simulink model "IEEE_9bus"  (R2023b)
settings: Solver=ode23tb  StartTime=0.0  StopTime=1  FixedStep=Ts  RelTol=1e-3
values from neighbouring files (symbols this model uses):
  N = 1    [IEEE_9bus_calc.m]
  Ts = 50e-6    (= 5e-05)    [IEEE_9bus_calc.m]
  Ws = 2*pi*f    (= 376.991118431)    [IEEE_9bus_calc.m]
undefined symbols (not defined in the file or in its folder): D1, Delta, DiscIntNeverNeededParam, SM, SYS
libraries: spsLoadFlowBusLib x9, spsabctodq0Lib x7, spsThreePhasePISectionLineLib x6, spsExcitationSystemLib x6, spsGenericPowerSystemStabilizerLib x6, spsHydraulicTurbineandGovernorLib x6, spsMultiBandPowerSystemStabilizerLib x6, spsThreePhaseVIMeasurementLib x5, spsThreePhaseSeriesRLCLoadLib x4, DQN_Lib x3, spsGroundLib x3, spsThreePhaseParallelRLCBranchLib x3
(part 2 of 3)

== system IEEE_9bus/ABsel ==
  In1 : Inport
  Demux : Demux  Outputs=3
  Mux : Mux  Inputs=3
  Subtract : Sum  Inputs=--
  Out1 : Outport
  wires:
  In1/1 -> Demux/1
  Demux/1 -> Subtract/1, Mux/1
  Mux/1 -> Out1/1
  Demux/2 -> Subtract/2, Mux/2
  Subtract/1 -> Mux/3

== system IEEE_9bus/ABsel1 ==
  In1 : Inport
  Demux : Demux  Outputs=3
  Mux : Mux  Inputs=3
  Subtract : Sum  Inputs=--
  Out1 : Outport
  wires:
  In1/1 -> Demux/1
  Demux/1 -> Subtract/1, Mux/1
  Mux/1 -> Out1/1
  Demux/2 -> Subtract/2, Mux/2
  Subtract/1 -> Mux/3

== system IEEE_9bus/ABsel2 ==
  In1 : Inport
  Demux : Demux  Outputs=3
  Mux : Mux  Inputs=3
  Subtract : Sum  Inputs=--
  Out1 : Outport
  wires:
  In1/1 -> Demux/1
  Demux/1 -> Subtract/1, Mux/1
  Mux/1 -> Out1/1
  Demux/2 -> Subtract/2, Mux/2
  Subtract/1 -> Mux/3

== system IEEE_9bus/ABsel3 ==
  In1 : Inport
  Demux : Demux  Outputs=3
  Mux : Mux  Inputs=2
  Subtract : Sum  Inputs=+-
  Subtract1 : Sum  Inputs=+-
  Out1 : Outport
  wires:
  In1/1 -> Demux/1
  Mux/1 -> Out1/1
  Demux/1 -> Subtract/1
  Demux/2 -> Subtract1/1, Subtract/2
  Subtract/1 -> Mux/1
  Subtract1/1 -> Mux/2
  Demux/3 -> Subtract1/2

== system IEEE_9bus/ABsel4 ==
  In1 : Inport
  Demux : Demux  Outputs=2
  Mux : Mux  Inputs=3
  Subtract : Sum  Inputs=--
  Out1 : Outport
  wires:
  In1/1 -> Demux/1
  Demux/1 -> Subtract/1, Mux/1
  Mux/1 -> Out1/1
  Demux/2 -> Mux/2, Subtract/2
  Subtract/1 -> Mux/3

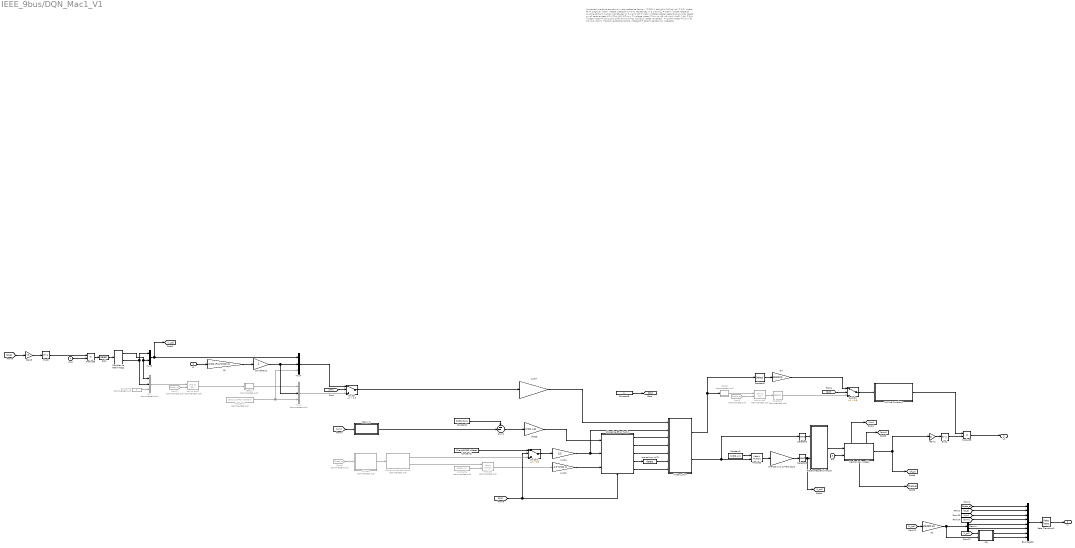
== system IEEE_9bus/DQN_Mac1_V1 ==
  note: Implement  machine equations in rotor reference frame:
      |   v = [R]*i + dphi/dt + [W]*phi
      | phi = [L]*i
      |
      | where:
      | [R] = diagonal matrix (nState,nState)of winding resistances in d q axis
      | [L] = matrix (nSate,nState)of winding self and mutual inductances in d q axis
      | [W] = matrix (nState,nState) depending on rotor speed wr,
      |       all zeros except W(1,2)=wr  W(2,1)=-wr
      |
      |   v = voltage vector      = [vq   vd   vfd   vkd   vkq1   (vkq2)  ]'
      | phi = flux linkage vector = [phiq phid phifd phikd phikq1 (phikq2)]' (state variables)
      |   i = current vector      = [iq   id   ifd   ikd   ikq1   (ikq2)  ]'
      |
      | if RotorType=Salient-Pole, nState=5
      | if RotorType=Round,        nState=6
  Vs_C : Inport
  Vf : Inport  Port=2
  Pm : Inport  Port=3
  1_Vb1 : Gain  Gain=-0.5*SMRD.Ib  SaturateOnIntegerOverflow=on  OutDataTypeStr=Inherit: Same as input  ParamDataTypeStr=Inherit: Same as input
  1_Vb4 : Gain  Gain=1/3  SaturateOnIntegerOverflow=on  OutDataTypeStr=Inherit: Same as input  ParamDataTypeStr=Inherit: Same as input
  1_Vb7 : Gain  Gain=SMRD.web/SMRD.Vb  SaturateOnIntegerOverflow=on  OutDataTypeStr=Inherit: Same as input  ParamDataTypeStr=Inherit: Same as input
  ABsel2 : Subsystem  Commented=on
  ABsel3 : Subsystem  Commented=on
  Bus Creator : BusCreator  Inputs=8
  Complex to Real-Imag1 : ComplexToRealImag
  Constant : Constant  Commented=on  Value=zeros(1,SMRD.nState-3)
  Constant1 : Constant  Value=SMRD.RLinv
  Constant2 : Constant  Value=3*eye(SMRD.nState)
  Constant4 : Constant  Commented=on  Value=SMRD.Linv
  Constant5 : Constant  Commented=on  Value=0
  Constant7 : Constant  Value=SMRD.Linv
  Constant8 : Constant
  Demux : Demux  Outputs=2
  Discretize BE or Tustin : Subsystem
      settings: PortSchema="{\"entries\":[{\"content\":{\"sides\":[{\"content\":{\"connectorIds\":[\"In1\",\"In2\",\"In3\"]},\"type\":\"ConnectorPlacement.EquallySpacedRectSide\",\"uuid\":\"a6b8bc68-dacc-495a-bf9e-1715fd4ce50f\"},{\"content\":{\"connectorIds\":[\"Out1\",\"Out2\",\"Out3\",\"Out4\",\"Out5\"],\"side\":\"RIGHT\"},\"type\":\"ConnectorPlacement.EquallySpacedRectSide\",\"uuid\":\"950ac892-f5e8-4081-8a8f-99bab3dfce2c\"},{\"content\":{\"side\":\"TOP\"},\"type\":\"ConnectorPlacement.EquallySpacedRectSide\",\"uuid\":\"9af2ed0d-ba89-43cd-9977-15872ca13b39\"},{\"content\":{\"connectorIds\":[\"In4\"],\"side\":\"BOTTOM\"},\"type\":\"ConnectorPlacement.EquallySpacedRectSide\",\"uuid\":\"e70e144b-23c4-40ad-9fe1-8550fd976efc\"}]},\"type\":\"ConnectorPlacement.EquallySpacedConnector\",\"uuid\":\"50b9889c-6d2c-45b1-ad8f-98a7760fa0a3\"}],\"packageUris\":[\"http://schema.mathworks.com/mf0/Connector/R2020b\"],\"version\":\"1.0\"}"
  Electromagnetic Torque : Subsystem
  Exp2 : Math
  Exp3 : Math
  From3 : From  Commented=on  GotoTag=theta_e
  From5 : From  Commented=on  GotoTag=theta_e
  From8 : From  Commented=on  GotoTag=theta_e
  Gain2 : Gain  Gain=1i
  Gain3 : Gain  Gain=-1i
  Ihistory_Flux : Subsystem
  MATLAB Function2 : MATLAB Function  TreatAsAtomicUnit=on  mask{N=SMRD.N}
      mask prompts: N "Harmonic order:"
  Matrix W : Subsystem
      settings: LibrarySourceBlock=spsSynchronousMachineModel/Discrete robust/Matrix W
  Mechanical model1 : Subsystem
      settings: LibrarySourceBlock=spsSynchronousMachineModel/Discrete Pm input trapezoidal  PortSchema="{\"entries\":[{\"content\":{\"sides\":[{\"content\":{\"connectorIds\":[\"In1\",\"In2\"]},\"type\":\"ConnectorPlacement.EquallySpacedRectSide\",\"uuid\":\"2381534f-5abc-4a8d-aa04-ab974f15f8a1\"},{\"content\":{\"connectorIds\":[\"Out1\"],\"side\":\"RIGHT\"},\"type\":\"ConnectorPlacement.EquallySpacedRectSide\",\"uuid\":\"4b91f832-d568-486f-91ee-7f5a07d19f05\"},{\"content\":{\"connectorIds\":[\"Out3\",\"Out4\"],\"side\":\"TOP\"},\"type\":\"ConnectorPlacement.EquallySpacedRectSide\",\"uuid\":\"94f23016-8fd9-49f0-81e0-4b44cc2bc22e\"},{\"content\":{\"connectorIds\":[\"Out2\"],\"side\":\"BOTTOM\"},\"type\":\"ConnectorPlacement.EquallySpacedRectSide\",\"uuid\":\"caf2a10e-4688-4978-a259-17b5afc46c0a\"}]},\"type\":\"ConnectorPlacement.EquallySpacedConnector\",\"uuid\":\"5998548e-4f7b-436e-b4ae-37de4e285cc4\"}],\"packageUris\":[\"http://schema.mathworks.com/mf0/Connector/R2020b\"],\"version\":\"1.0\"}"
  Mux : Mux  Commented=on  Inputs=3
  Mux1 : Mux  Commented=on  Inputs=[2 1 SMRD.nState-3]
  Mux3 : Mux  Inputs=2
  Mux4 : Mux  Inputs=[2 1 SMRD.nState-3]
  N1 : Gain  Gain=SMRD.Vfnp*SMRD.Vb  SaturateOnIntegerOverflow=on  OutDataTypeStr=Inherit: Same as input  ParamDataTypeStr=Inherit: Same as input
  N2 : Gain  Gain=1/SMRD.Vb  SaturateOnIntegerOverflow=on  OutDataTypeStr=Inherit: Same as input  ParamDataTypeStr=Inherit: Same as input
  PQ : Subsystem  AncestorBlock=spsSynchronousMachineModel/Discrete robust/Machine Measurements/PQ
  Product2 : Product  Multiplication=Matrix(*)  SaturateOnIntegerOverflow=on  OutDataTypeStr=Inherit: Same as first input
  Product4 : Product  Commented=on  Multiplication=Matrix(*)  SaturateOnIntegerOverflow=on  OutDataTypeStr=Inherit: Same as first input
  Product5 : Product
  Product6 : Product
  Rate Transition2 : RateTransition  Deterministic=off  OutPortSampleTime=Ts
  SM.VfGain1 : Gain
  Sel1 : Selector  NumberOfDimensions=2  InputPortWidth=3  IndexOptions=Index vector (dialog),Index vector (dialog)  Indices=1,2  OutputSizes=1
  Selector1 : Selector  Commented=on  InputPortWidth=3  IndexOptions=Index vector (dialog)  Indices=[1 2]  OutputSizes=1
  Selector2 : Selector  InputPortWidth=SMRD.nState  IndexOptions=Index vector (dialog)  Indices=[1 2]  OutputSizes=1
  Selector3 : Selector  InputPortWidth=SMRD.nState  IndexOptions=Index vector (dialog)  Indices=[1 2]  OutputSizes=1
  Selector5 : Selector  InputPortWidth=2  IndexOptions=Index vector (dialog)  Indices=[2 1]  OutputSizes=1
  Sum1 : Sum  Inputs=--|  SaturateOnIntegerOverflow=on
  Switch : Switch  Criteria=u2 > Threshold  Threshold=0.5  SaturateOnIntegerOverflow=off  InputSameDT=off
  Switch1 : Switch  Criteria=u2 > Threshold  Threshold=0.5  SaturateOnIntegerOverflow=off  InputSameDT=off
  Switch3 : Switch  Criteria=u2 > Threshold  Threshold=0.5  SaturateOnIntegerOverflow=off  InputSameDT=off
  abc to dq transformation : Subsystem  Commented=on
      settings: LibrarySourceBlock=|
      | spsSynchronousMachineModel/Discrete robust/abc to dq
      | transformation
  abc to dq0 : spsabctodq0Lib/abc to dq0  Commented=on  Alignment=90 degrees behind phase A axis
  change Iq Id current signs : Gain  Gain=SMRD.IqdSign
  dq0 to abc1 : spsdq0toabcLib/dq0 to abc  Commented=on  Alignment=90 degrees behind phase A axis
  ib4 : Gain  Gain=SMRD.Ib  SaturateOnIntegerOverflow=on  OutDataTypeStr=Inherit: Same as input  ParamDataTypeStr=Inherit: Same as input
  last column of D : Selector  NumberOfDimensions=2  InputPortWidth=3  IndexOptions=Index vector (dialog),Index vector (dialog)  Indices=[1:SMRD.nState],3  OutputSizes=1,1
  sin,cos : Subsystem  Commented=on
      settings: LibrarySourceBlock=spsSynchronousMachineModel/Discrete robust/sin,cos
  wbase : Gain  Gain=SMRD.web
  I_C : Outport  VectorParamsAs1DForOutWhenUnconnected=off
  m : Outport  Port=2  VectorParamsAs1DForOutWhenUnconnected=off
  wires:
  Vs_C/1 -> Product6/2  "vd,vq"
  sin,cos/1(sin,cos) -> abc to dq transformation/1(sin,cos)
  1_Vb1/1 -> Discretize BE or Tustin/3(C)
  last column of D/1 -> Ihistory_Flux/6(D(:,3))
  Discretize BE or Tustin/1(Ad) -> Ihistory_Flux/3(Ad)
  Discretize BE or Tustin/4(Dd) -> last column of D/1
  Electromagnetic Torque/1(Te) -> Mechanical model1/1(Te)
  Product2/1 -> change Iq Id current signs/1
  wbase/1 -> Discretize BE or Tustin/1(A)
  Discretize BE or Tustin/5(inv(I_Ts/2*A)) -> Ihistory_Flux/7(inv())
  Discretize BE or Tustin/2(Bd) -> Ihistory_Flux/4(Bd)
  Constant4/1 -> Product4/2  "Linv"
  Matrix W/1("[W]") -> Sum1/2
  Sum1/1 -> wbase/1  "A"
  Product4/1 -> 1_Vb1/1
  Ihistory_Flux/2(phi) -> Product2/2, Selector2/1
  Mechanical model1/2(theta_e) -> [theta_e]
  Mechanical model1/3(we) -> [wm]
  Pm/1 -> Mechanical model1/2(input)
  Constant7/1 -> Product2/1  "Linv"
  Constant2/1 -> Switch1/1
  ABsel3/1(Out1) -> Mux1/1
  Mux1/1 -> Switch/3  "u"
  Constant1/1 -> Sum1/1
  Vf/1 -> N1/1  "Vfd"
  Constant/1 -> Mux1/3, Mux4/3
  SM.VfGain1/1 -> Mux4/2, Mux1/2
  Mux4/1 -> Switch/1  "u"
  N1/1 -> SM.VfGain1/1  "Vfd"
  dq0 to abc1/1 -> ABsel3/1(v)
  abc to dq transformation/2(Ti (2x2)) -> Product4/1
  Switch1/1 -> 1_Vb4/1  "u"
  Ihistory_Flux/1(Ihyst) -> Selector5/1, ABsel2/1(v)  "I(k) = Linv*phi"
  MATLAB Function2/1(Vs_c) -> Product5/1
  Exp2/1 -> Product5/2
  Gain2/1 -> Exp2/1
  Switch/1 -> 1_Vb7/1
  Gain3/1 -> Exp3/1
  [dt_e] -> Gain3/1
  Product6/1 -> Sel1/1
  Exp3/1 -> Product6/1
  Sel1/1 -> Complex to Real-Imag1/1
  Mechanical model1/1(dtheta_e) -> [dt_e], Gain2/1
  Complex to Real-Imag1/2 -> Mux3/1, Mux/2
  Complex to Real-Imag1/1 -> Mux/1, Mux3/2
  Mux3/1 -> [v_qd], Mux4/1
  Switch3/1 -> MATLAB Function2/1(Vdq_vec)
  Mux/1 -> dq0 to abc1/1
  From3/1 -> dq0 to abc1/2
  Constant5/1 -> Mux/3
  1_Vb7/1 -> Ihistory_Flux/1(u)  "u"
  [SW] -> Switch/2
  Constant8/1 -> [SW]
  [SW] -> Switch1/2, Discretize BE or Tustin/4(SW)
  abc to dq transformation/1(Tv (nx3)) -> Switch1/3
  Selector1/1 -> Switch3/3  "Linv"
  [SW] -> Switch3/2
  Selector5/1 -> ib4/1
  abc to dq0/1 -> Selector1/1
  ABsel2/1(I) -> abc to dq0/1
  ib4/1 -> Switch3/1
  From5/1 -> abc to dq0/2
  Product5/1 -> I_C/1
  1_Vb4/1 -> Ihistory_Flux/2(B), Discretize BE or Tustin/2(B)
  [wm] -> Matrix W/1(wr)
  From8/1 -> sin,cos/1(theta)
  Discretize BE or Tustin/3(Cd) -> Ihistory_Flux/5(Cd)
  Bus Creator/1 -> Rate Transition2/1
  [theta_e] -> Bus Creator/1  "Rotor electrical angle  theta (rad)"
  [dt_e] -> Bus Creator/2  "Rotor angle deviation  d_theta (rad)"
  [wm] -> Bus Creator/3  "Rotor speed  wm  (pu)"
  Rate Transition2/1 -> m/1
  [v_qd] -> N2/1
  [i_qd] -> PQ/1(Iqd)
  PQ/1(Peo) -> Bus Creator/7  "Output active power   Peo (pu)"
  PQ/2(Qeo) -> Bus Creator/8  "Output reactive power  Qeo (pu)"
  Mechanical model1/4(dwe) -> [dwm]
  [dwm] -> Bus Creator/4  "Rotor speed deviation  dw (pu)"
  change Iq Id current signs/1 -> Selector3/1
  Selector3/1 -> [i_qd], Electromagnetic Torque/2(iqd)
  Selector2/1 -> Electromagnetic Torque/1(phiqd)
  N2/1 -> PQ/2(Vqd), Demux/1  "Vfd"
  Demux/1 -> Bus Creator/5  "Stator voltage  vq (pu)"
  Demux/2 -> Bus Creator/6  "Stator voltage  vd (pu)"

== system IEEE_9bus/Demux_DQNc_Mat ==
  In1 : Inport
  Sel1 : Selector  NumberOfDimensions=2  InputPortWidth=3  IndexOptions=Index vector (dialog),Select all  Indices=1:3, 1  OutputSizes=1
  Sel2 : Selector  NumberOfDimensions=2  InputPortWidth=3  IndexOptions=Index vector (dialog),Select all  Indices=4:6, 1  OutputSizes=1
  Sel3 : Selector  NumberOfDimensions=2  InputPortWidth=3  IndexOptions=Index vector (dialog),Select all  Indices=7:9, 1  OutputSizes=1
  Out1 : Outport
  Out2 : Outport  Port=2
  Out3 : Outport  Port=3
  wires:
  In1/1 -> Sel1/1, Sel2/1, Sel3/1
  Sel1/1 -> Out1/1
  Sel2/1 -> Out2/1
  Sel3/1 -> Out3/1

== system IEEE_9bus/Demux_DQNc_Mat2 ==
  In1 : Inport
  Sel1 : Selector  NumberOfDimensions=2  InputPortWidth=3  IndexOptions=Index vector (dialog),Select all  Indices=1:3, 1  OutputSizes=1
  Sel2 : Selector  NumberOfDimensions=2  InputPortWidth=3  IndexOptions=Index vector (dialog),Select all  Indices=4:6, 1  OutputSizes=1
  Sel3 : Selector  NumberOfDimensions=2  InputPortWidth=3  IndexOptions=Index vector (dialog),Select all  Indices=7:9, 1  OutputSizes=1
  Out1 : Outport
  Out2 : Outport  Port=2
  Out3 : Outport  Port=3
  wires:
  In1/1 -> Sel1/1, Sel2/1, Sel3/1
  Sel1/1 -> Out1/1
  Sel2/1 -> Out2/1
  Sel3/1 -> Out3/1

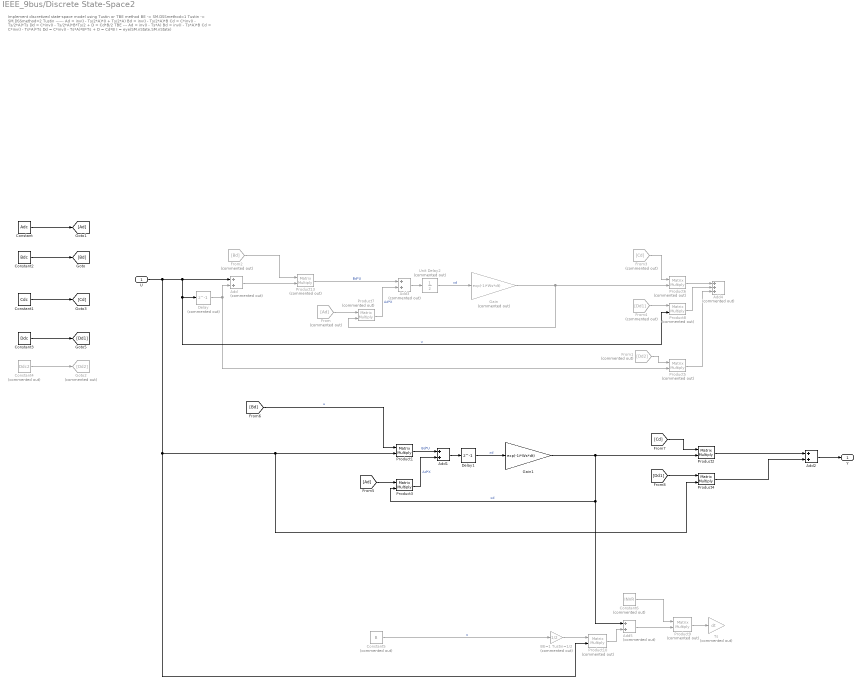
== system IEEE_9bus/Discrete State-Space2 ==
  note: Implement discretized state-space model using Tustin or TBE method
      |
      | BE      -> SM.DSSmethod=1
      | Tustin  -> SM.DSSmethod=2
      |
      |
      | Tustin
      | ------
      | Ad = inv(I - Ts/2*A)*(I + Ts/2*A)
      | Bd = inv(I - Ts/2*A)*B
      | Cd = C*inv(I - Ts/2*A)*Ts
      | Dd = C*inv(I - Ts/2*A)*B*Ts/2  + D  =  Cd*B/2
      |
      | TBE
      | ---
      | Ad = inv(I - Ts*A)
      | Bd = inv(I - Ts*A)*B
      | Cd = C*inv(I - Ts*A)*Ts
      | Dd = C*inv(I - Ts*A)*B*Ts  + D  =  Cd*B
      |
      | I = eye(SM.nState,SM.nState)
  U : Inport
  Add : Sum  Commented=on
  Add1 : Sum
  Add2 : Sum
  Add3 : Sum  Commented=on
  Add4 : Sum  Commented=on  Inputs=+++
  Add5 : Sum  Commented=on
  BE=1 Tustin=1/2 : Gain  Commented=on  Gain=1/2
  Constant : Constant  Value=Adc
  Constant1 : Constant  Value=Cdc
  Constant2 : Constant  Value=Bdc
  Constant3 : Constant  Value=Ddc
  Constant4 : Constant  Commented=on  Value=Ddc2
  Constant5 : Constant  Commented=on  Value=B
  Constant6 : Constant  Commented=on  Value=INVR
  Delay : Delay  Commented=on  DelayLength=1  SampleTime=dt
  Delay1 : Delay  DelayLength=1  InitialCondition=InitVec_c  SampleTime=dt
  From : From  Commented=on  GotoTag=Ad
  From1 : From  Commented=on  GotoTag=Dd2
  From2 : From  Commented=on  GotoTag=Bd
  From3 : From  Commented=on  GotoTag=Cd
  From4 : From  Commented=on  GotoTag=Dd1
  Gain : Gain  Commented=on  Gain=exp(-1i*Ws*dt)
  Gain1 : Gain  Gain=exp(-1i*Ws*dt)
  Goto2 : Goto  Commented=on  GotoTag=Dd2
  Product{1..4} (4 alike) : Product  Multiplication=Matrix(*)  SaturateOnIntegerOverflow=on  OutDataTypeStr=Inherit: Same as first input
  Product{5..10,13} (7 alike) : Product  Commented=on  Multiplication=Matrix(*)  SaturateOnIntegerOverflow=on  OutDataTypeStr=Inherit: Same as first input
  Ts : Gain  Commented=on  Gain=dt  SaturateOnIntegerOverflow=on  OutDataTypeStr=Inherit: Same as input  ParamDataTypeStr=Inherit: Same as input
  Unit Delay2 : UnitDelay  Commented=on  InitialCondition=(Cdc\InitVec_c)  SampleTime=dt  HasFrameUpgradeWarning=on
  Y : Outport
  wires:
  Constant4/1 -> Goto2/1
  Constant3/1 -> [Dd1]
  Constant1/1 -> [Cd]
  Constant2/1 -> [Bd]
  Constant/1 -> [Ad]
  From1/1 -> Product5/1
  Product5/1 -> Add4/3
  Product8/1 -> Add4/2
  From/1 -> Product7/1
  From4/1 -> Product8/1
  From2/1 -> Product13/1
  Product13/1 -> Add3/1  "Bd*U"
  Product7/1 -> Add3/2  "Ad*X"
  Add/1 -> Product13/2
  Product6/1 -> Add4/1
  Unit Delay2/1 -> Gain/1  "xd"
  From3/1 -> Product6/1
  Delay/1 -> Product5/2, Add/2
  Add3/1 -> Unit Delay2/1
  Gain/1 -> Product7/2, Product6/2
  Product1/1 -> Add1/1  "Bd*U"
  Product2/1 -> Add2/1
  [Dd1] -> Product4/1
  Product4/1 -> Add2/2
  [Bd] -> Product1/1  "u"
  Product3/1 -> Add1/2  "Ad*X"
  [Cd] -> Product2/1
  Delay1/1 -> Gain1/1  "xd"
  Add1/1 -> Delay1/1
  [Ad] -> Product3/1
  Constant5/1 -> BE=1 Tustin=1/2/1  "u"
  Product9/1 -> Ts/1
  Constant6/1 -> Product9/1
  Add5/1 -> Product9/2
  U/1 -> Product10/2, Product4/2, Product1/2, Add/1, Product8/2, Delay/1  "u"
  BE=1 Tustin=1/2/1 -> Product10/1
  Product10/1 -> Add5/2
  Gain1/1 -> Product3/2, Add5/1, Product2/2  "xd"
  Add2/1 -> Y/1

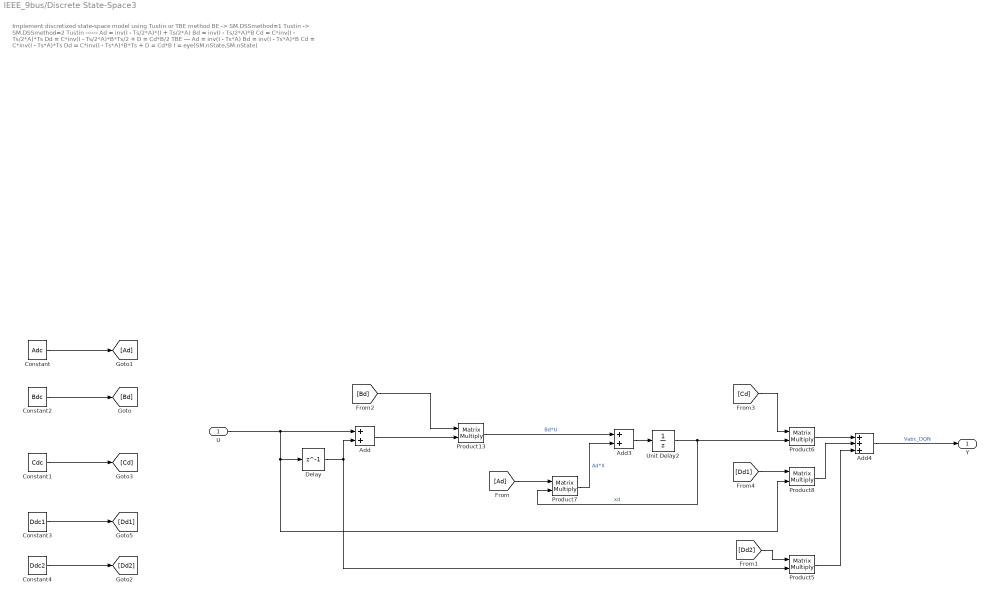
== system IEEE_9bus/Discrete State-Space3 ==
  note: Implement discretized state-space model using Tustin or TBE method
      |
      | BE      -> SM.DSSmethod=1
      | Tustin  -> SM.DSSmethod=2
      |
      |
      | Tustin
      | ------
      | Ad = inv(I - Ts/2*A)*(I + Ts/2*A)
      | Bd = inv(I - Ts/2*A)*B
      | Cd = C*inv(I - Ts/2*A)*Ts
      | Dd = C*inv(I - Ts/2*A)*B*Ts/2  + D  =  Cd*B/2
      |
      | TBE
      | ---
      | Ad = inv(I - Ts*A)
      | Bd = inv(I - Ts*A)*B
      | Cd = C*inv(I - Ts*A)*Ts
      | Dd = C*inv(I - Ts*A)*B*Ts  + D  =  Cd*B
      |
      | I = eye(SM.nState,SM.nState)
  U : Inport
  Add : Sum
  Add3 : Sum
  Add4 : Sum  Inputs=+++
  Constant : Constant  Value=Adc
  Constant1 : Constant  Value=Cdc
  Constant2 : Constant  Value=Bdc
  Constant3 : Constant  Value=Ddc1
  Constant4 : Constant  Value=Ddc2
  Delay : Delay  DelayLength=1  SampleTime=Ts
  Product{5..8,13} (5 alike) : Product  Multiplication=Matrix(*)  SaturateOnIntegerOverflow=on  OutDataTypeStr=Inherit: Same as first input
  Unit Delay2 : UnitDelay  InitialCondition=InitVec_c  SampleTime=dt  HasFrameUpgradeWarning=on
  Y : Outport
  wires:
  Constant4/1 -> [Dd2]
  Constant3/1 -> [Dd1]
  Constant1/1 -> [Cd]
  Constant2/1 -> [Bd]
  Constant/1 -> [Ad]
  Add4/1 -> Y/1  "Vabc_DQN"
  [Dd2] -> Product5/1
  Product5/1 -> Add4/3
  Product8/1 -> Add4/2
  [Ad] -> Product7/1
  [Dd1] -> Product8/1
  U/1 -> Add/1, Product8/2, Delay/1
  [Bd] -> Product13/1
  Product13/1 -> Add3/1  "Bd*U"
  Product7/1 -> Add3/2  "Ad*X"
  Add/1 -> Product13/2
  Product6/1 -> Add4/1
  Unit Delay2/1 -> Product7/2, Product6/2  "xd"
  [Cd] -> Product6/1
  Delay/1 -> Product5/2, Add/2
  Add3/1 -> Unit Delay2/1

== system IEEE_9bus/MatMux1 ==
  In1 : Inport
  In2 : Inport  Port=2
  In3 : Inport  Port=3
  Mux : Concatenate  NumInputs=3  Mode=Multidimensional array
  Out1 : Outport
  wires:
  In1/1 -> Mux/1
  In2/1 -> Mux/2
  In3/1 -> Mux/3
  Mux/1 -> Out1/1

== system IEEE_9bus/MatMux2 ==
  In1 : Inport
  In2 : Inport  Port=2
  In3 : Inport  Port=3
  Mux : Concatenate  NumInputs=3  Mode=Multidimensional array
  Out1 : Outport
  wires:
  In1/1 -> Mux/1
  In2/1 -> Mux/2
  In3/1 -> Mux/3
  Mux/1 -> Out1/1

== system IEEE_9bus/MatMux3 ==
  In1 : Inport
  In2 : Inport  Port=2
  In3 : Inport  Port=3
  Mux : Concatenate  NumInputs=3  Mode=Multidimensional array
  Out1 : Outport
  wires:
  In1/1 -> Mux/1
  In2/1 -> Mux/2
  In3/1 -> Mux/3
  Mux/1 -> Out1/1

== system IEEE_9bus/SS_DelayPrediction ==
  in : Inport
  F2 : Gain  Gain=2  SaturateOnIntegerOverflow=on  OutDataTypeStr=Inherit: Same as input  ParamDataTypeStr=Inherit: Same as input
  Sum1 : Sum  Inputs=+-  InputSameDT=on  SaturateOnIntegerOverflow=on  OutDataTypeStr=Inherit: Same as first input
  dw_delay : UnitDelay  InitialCondition=Zpnz_old  SampleTime=Ts  HasFrameUpgradeWarning=on
  dw_predict : UnitDelay  InitialCondition=Zpnz_old  SampleTime=Ts  HasFrameUpgradeWarning=on
  dw : Outport  VectorParamsAs1DForOutWhenUnconnected=off
  wires:
  Sum1/1 -> dw/1
  F2/1 -> Sum1/1
  dw_predict/1 -> Sum1/2
  in/1 -> dw_delay/1
  dw_delay/1 -> F2/1, dw_predict/1

== system IEEE_9bus/Subsystem ==
  cte1 : Constant
  cte2 : Constant  Value=2
  cte3 : Constant  Value=0
  Generic : Outport  VectorParamsAs1DForOutWhenUnconnected=off
  Multiband : Outport  Port=2  VectorParamsAs1DForOutWhenUnconnected=off
  No PSS : Outport  Port=3  VectorParamsAs1DForOutWhenUnconnected=off
  wires:
  cte1/1 -> Generic/1
  cte2/1 -> Multiband/1
  cte3/1 -> No PSS/1

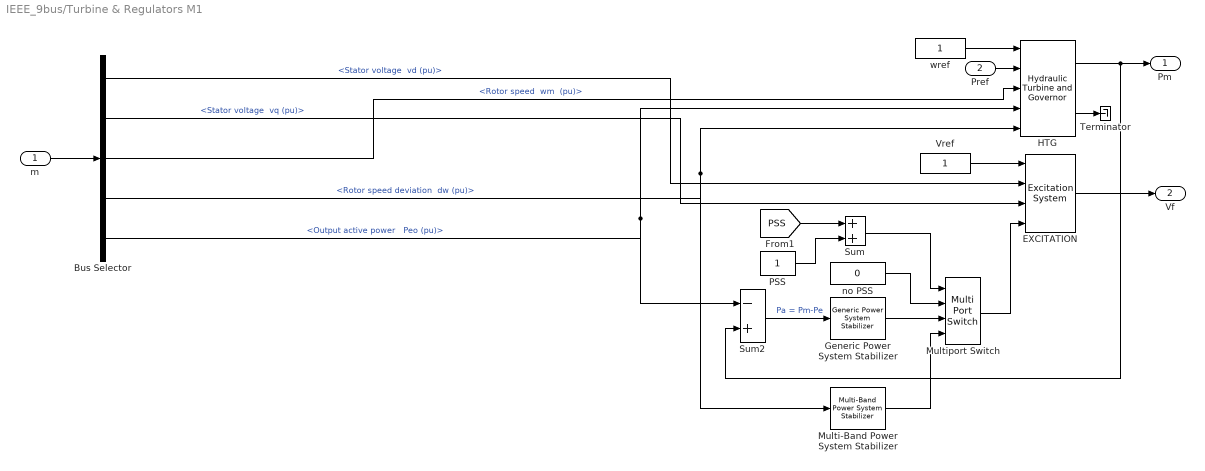
== system IEEE_9bus/Turbine & Regulators M1 ==
  m : Inport
  Pref : Inport  Port=2
  Bus Selector : BusSelector  OutputSignals="dq0 components.Stator voltage  vd (pu),dq0 components.Stator voltage  vq (pu),Mechanical.Rotor speed  wm  (pu),Mechanical.Rotor speed deviation  dw (pu),Output active power   Peo (pu)"
  EXCITATION : spsExcitationSystemLib/Excitation System  tr=20e-3  reg=[ 200, 0.001 ]  exc=[ 1, 0 ]  tgr=[ 0, 0 ]  damp=[ 0.001, 0.1 ]  sat=[ 0, 0 ]  lim="[ 0,  7, 0 ]"  v0=[1 1.5789]
      settings: LibrarySourceBlock=sps_lib/Electrical Machines/Synchronous Machine Control/Excitation System
  Generic Power System Stabilizer : spsGenericPowerSystemStabilizerLib/Generic Power System Stabilizer  Tsensor=15e-3  K=2  Twashout=0.7  Tleadlag1="[60e-3  0.5]"  Tleadlag2=[0 0]  VSlimits=[-0.15 0.15]  Vinit=0  Plot_On=off  MagdB_On=on  FreqRange=logspace(-2,2,500)
      settings: LibrarySourceBlock=|
      | sps_lib/Electrical Machines/Synchronous Machine Control/Generic
      | Power System Stabilizer
  HTG : spsHydraulicTurbineandGovernorLib/Hydraulic Turbine and Governor  sm="[ 10/3  0.07 ]"  gate="[  0.01  0.97518  -0.1  0.1 ]"  reg="[  0.05  1.163  0.105  0  0.01  ]"  hyd="[  0  2.67  ]"  dref=0  po=0.65844
      settings: LibrarySourceBlock=|
      | sps_lib/Electrical Machines/Synchronous Machine Control/Hydraulic Turbine
      | and Governor
  Multi-Band Power System Stabilizer : spsMultiBandPowerSystemStabilizerLib/Multi-Band Power System Stabilizer  OperationMode=Simplified settings  Kg=1.0  GL=[0.025 5]  GI=[0.8 25]  GH=[12.0 145]  GLd=[66 66 9.4]  TcLF=[1.667 2 0 0 0 0 2 2.4 0 0 0 0 1 1]  GId=[66 66 47.6]  TcIF=[1 1 0.25 0.3 0 0 1 1 0.3 0.36 0 0 0 0]  GHd=[66 66 233]  TcHF="[0.01 0.012 0 0 0 0  0.012 0.0144 0 0 0 0 1 1]"  LIM=[.075 .15 .15 .15]  Plot_On=off  MagdB_On=off  FreqRange=logspace(-2,2,500)
      settings: LibrarySourceBlock=|
      | sps_lib/Electrical Machines/Synchronous Machine Control/Multi-Band
      | Power System Stabilizer
  Multiport Switch : MultiPortSwitch  InputSameDT=off
  PSS : Constant
  Sum : Sum  SaturateOnIntegerOverflow=on
  Sum2 : Sum  Inputs=-+  InputSameDT=on  SaturateOnIntegerOverflow=on  OutDataTypeStr=Inherit: Same as first input
  Terminator : Terminator
  Vref : Constant
  no PSS : Constant  Value=0
  wref : Constant
  Pm : Outport  InitialOutput=0  VectorParamsAs1DForOutWhenUnconnected=off
  Vf : Outport  Port=2  InitialOutput=0  VectorParamsAs1DForOutWhenUnconnected=off
  wires:
  PSS/1 -> Sum/2
  [PSS] -> Sum/1
  HTG/2 -> Terminator/1
  Vref/1 -> EXCITATION/1
  m/1 -> Bus Selector/1
  Bus Selector/4 -> Multi-Band Power System Stabilizer/1, HTG/5  "<Rotor speed deviation  dw (pu)>"
  Bus Selector/5 -> Sum2/1, HTG/4  "<Output active power   Peo (pu)>"
  Bus Selector/3 -> HTG/3  "<Rotor speed  wm  (pu)>"
  Pref/1 -> HTG/2
  wref/1 -> HTG/1
  HTG/1 -> Pm/1, Sum2/2
  Bus Selector/2 -> EXCITATION/3  "<Stator voltage  vq (pu)>"
  EXCITATION/1 -> Vf/1
  Bus Selector/1 -> EXCITATION/2  "<Stator voltage  vd (pu)>"
  Sum2/1 -> Generic Power System Stabilizer/1  "Pa = Pm-Pe"
  Generic Power System Stabilizer/1 -> Multiport Switch/3
  Multi-Band Power System Stabilizer/1 -> Multiport Switch/4
  no PSS/1 -> Multiport Switch/2
  Sum/1 -> Multiport Switch/1
  Multiport Switch/1 -> EXCITATION/4

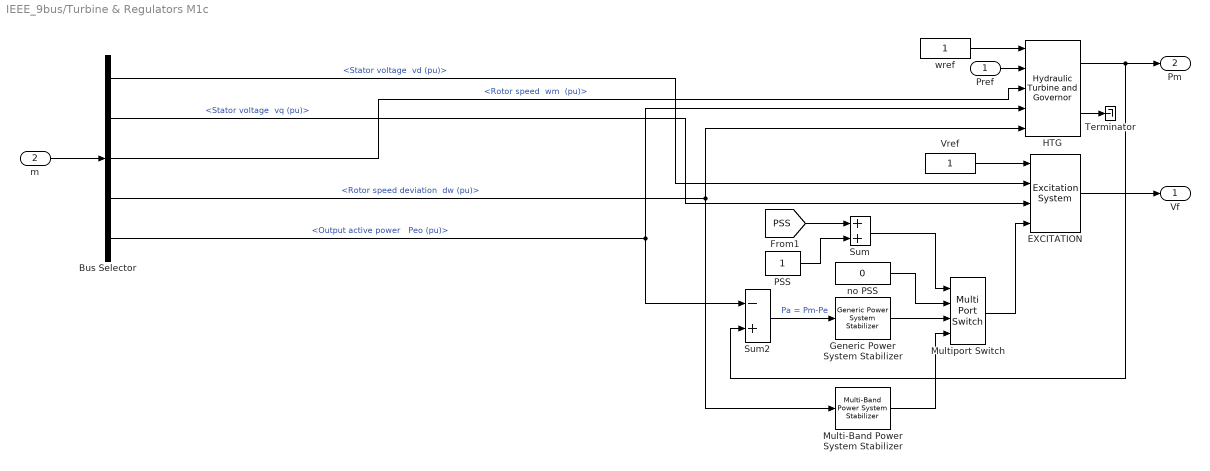
== system IEEE_9bus/Turbine & Regulators M1c ==
  Pref : Inport
  m : Inport  Port=2
  Bus Selector : BusSelector  OutputSignals="Stator voltage  vd (pu),Stator voltage  vq (pu),Rotor speed  wm  (pu),Rotor speed deviation  dw (pu),Output active power   Peo (pu)"
  EXCITATION : spsExcitationSystemLib/Excitation System  tr=20e-3  reg=[ 200, 0.001 ]  exc=[ 1, 0 ]  tgr=[ 0, 0 ]  damp=[ 0.001, 0.1 ]  sat=[ 0, 0 ]  lim="[ 0,  7, 0 ]"  v0=[1 1.5789]
      settings: LibrarySourceBlock=sps_lib/Electrical Machines/Synchronous Machine Control/Excitation System
  Generic Power System Stabilizer : spsGenericPowerSystemStabilizerLib/Generic Power System Stabilizer  Tsensor=15e-3  K=2  Twashout=0.7  Tleadlag1="[60e-3  0.5]"  Tleadlag2=[0 0]  VSlimits=[-0.15 0.15]  Vinit=0  Plot_On=off  MagdB_On=on  FreqRange=logspace(-2,2,500)
      settings: LibrarySourceBlock=|
      | sps_lib/Electrical Machines/Synchronous Machine Control/Generic
      | Power System Stabilizer
  HTG : spsHydraulicTurbineandGovernorLib/Hydraulic Turbine and Governor  sm="[ 10/3  0.07 ]"  gate="[  0.01  0.97518  -0.1  0.1 ]"  reg="[  0.05  1.163  0.105  0  0.01  ]"  hyd="[  0  2.67  ]"  dref=0  po=0.65844
      settings: LibrarySourceBlock=|
      | sps_lib/Electrical Machines/Synchronous Machine Control/Hydraulic Turbine
      | and Governor
  Multi-Band Power System Stabilizer : spsMultiBandPowerSystemStabilizerLib/Multi-Band Power System Stabilizer  OperationMode=Simplified settings  Kg=1.0  GL=[0.025 5]  GI=[0.8 25]  GH=[12.0 145]  GLd=[66 66 9.4]  TcLF=[1.667 2 0 0 0 0 2 2.4 0 0 0 0 1 1]  GId=[66 66 47.6]  TcIF=[1 1 0.25 0.3 0 0 1 1 0.3 0.36 0 0 0 0]  GHd=[66 66 233]  TcHF="[0.01 0.012 0 0 0 0  0.012 0.0144 0 0 0 0 1 1]"  LIM=[.075 .15 .15 .15]  Plot_On=off  MagdB_On=off  FreqRange=logspace(-2,2,500)
      settings: LibrarySourceBlock=|
      | sps_lib/Electrical Machines/Synchronous Machine Control/Multi-Band
      | Power System Stabilizer
  Multiport Switch : MultiPortSwitch  InputSameDT=off
  PSS : Constant
  Sum : Sum  SaturateOnIntegerOverflow=on
  Sum2 : Sum  Inputs=-+  InputSameDT=on  SaturateOnIntegerOverflow=on  OutDataTypeStr=Inherit: Same as first input
  Terminator : Terminator
  Vref : Constant
  no PSS : Constant  Value=0
  wref : Constant
  Vf : Outport  InitialOutput=0  VectorParamsAs1DForOutWhenUnconnected=off
  Pm : Outport  Port=2  InitialOutput=0  VectorParamsAs1DForOutWhenUnconnected=off
  wires:
  PSS/1 -> Sum/2
  [PSS] -> Sum/1
  HTG/2 -> Terminator/1
  Vref/1 -> EXCITATION/1
  m/1 -> Bus Selector/1
  Bus Selector/4 -> HTG/5, Multi-Band Power System Stabilizer/1  "<Rotor speed deviation  dw (pu)>"
  Bus Selector/5 -> HTG/4, Sum2/1  "<Output active power   Peo (pu)>"
  Bus Selector/3 -> HTG/3  "<Rotor speed  wm  (pu)>"
  Pref/1 -> HTG/2
  wref/1 -> HTG/1
  HTG/1 -> Pm/1, Sum2/2
  Bus Selector/2 -> EXCITATION/3  "<Stator voltage  vq (pu)>"
  EXCITATION/1 -> Vf/1
  Bus Selector/1 -> EXCITATION/2  "<Stator voltage  vd (pu)>"
  Sum2/1 -> Generic Power System Stabilizer/1  "Pa = Pm-Pe"
  Generic Power System Stabilizer/1 -> Multiport Switch/3
  Multi-Band Power System Stabilizer/1 -> Multiport Switch/4
  no PSS/1 -> Multiport Switch/2
  Sum/1 -> Multiport Switch/1
  Multiport Switch/1 -> EXCITATION/4

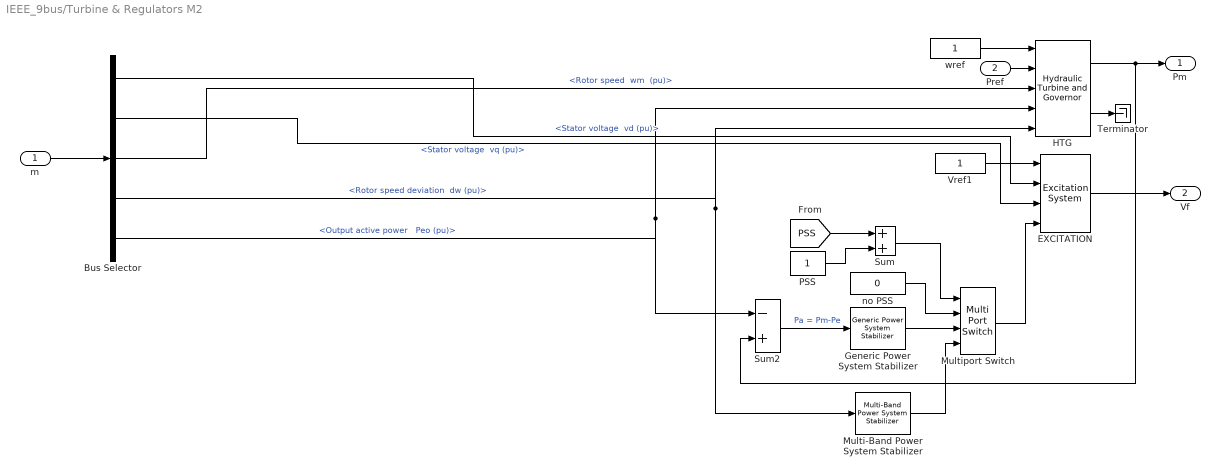
== system IEEE_9bus/Turbine & Regulators M2 ==
  m : Inport
  Pref : Inport  Port=2
  Bus Selector : BusSelector  OutputSignals="dq0 components.Stator voltage  vd (pu),dq0 components.Stator voltage  vq (pu),Mechanical.Rotor speed  wm  (pu),Mechanical.Rotor speed deviation  dw (pu),Output active power   Peo (pu)"
  EXCITATION : spsExcitationSystemLib/Excitation System  tr=20e-3  reg=[ 200, 0.001 ]  exc=[ 1, 0 ]  tgr=[ 0, 0 ]  damp=[ 0.001, 0.1 ]  sat=[ 0, 0 ]  lim="[ 0,  7, 0 ]"  v0=[1 1.5762]
      settings: LibrarySourceBlock=sps_lib/Electrical Machines/Synchronous Machine Control/Excitation System
  Generic Power System Stabilizer : spsGenericPowerSystemStabilizerLib/Generic Power System Stabilizer  Tsensor=15e-3  K=2  Twashout=0.7  Tleadlag1="[60e-3  0.5]"  Tleadlag2=[0 0]  VSlimits=[-0.15 0.15]  Vinit=0  Plot_On=off  MagdB_On=on  FreqRange=logspace(-2,2,500)
      settings: LibrarySourceBlock=|
      | sps_lib/Electrical Machines/Synchronous Machine Control/Generic
      | Power System Stabilizer
  HTG : spsHydraulicTurbineandGovernorLib/Hydraulic Turbine and Governor  sm="[ 10/3  0.07 ]"  gate="[  0.01  0.97518  -0.1  0.1 ]"  reg="[  0.05  1.163  0.105  0  0.01  ]"  hyd="[  0  2.67  ]"  dref=0  po=0.82708
      settings: LibrarySourceBlock=|
      | sps_lib/Electrical Machines/Synchronous Machine Control/Hydraulic Turbine
      | and Governor
  Multi-Band Power System Stabilizer : spsMultiBandPowerSystemStabilizerLib/Multi-Band Power System Stabilizer  OperationMode=Simplified settings  Kg=1.0  GL=[0.025 5]  GI=[0.8 25]  GH=[12.0 145]  GLd=[66 66 9.4]  TcLF=[1.667 2 0 0 0 0 2 2.4 0 0 0 0 1 1]  GId=[66 66 47.6]  TcIF=[1 1 0.25 0.3 0 0 1 1 0.3 0.36 0 0 0 0]  GHd=[66 66 233]  TcHF="[0.01 0.012 0 0 0 0  0.012 0.0144 0 0 0 0 1 1]"  LIM=[.075 .15 .15 .15]  Plot_On=off  MagdB_On=off  FreqRange=logspace(-2,2,500)
      settings: LibrarySourceBlock=|
      | sps_lib/Electrical Machines/Synchronous Machine Control/Multi-Band
      | Power System Stabilizer
  Multiport Switch : MultiPortSwitch  InputSameDT=off
  PSS : Constant
  Sum : Sum  SaturateOnIntegerOverflow=on
  Sum2 : Sum  Inputs=-+  InputSameDT=on  SaturateOnIntegerOverflow=on  OutDataTypeStr=Inherit: Same as first input
  Terminator : Terminator
  Vref1 : Constant
  no PSS : Constant  Value=0
  wref : Constant
  Pm : Outport  InitialOutput=0  VectorParamsAs1DForOutWhenUnconnected=off
  Vf : Outport  Port=2  InitialOutput=0  VectorParamsAs1DForOutWhenUnconnected=off
  wires:
  HTG/2 -> Terminator/1
  Vref1/1 -> EXCITATION/1
  m/1 -> Bus Selector/1
  Bus Selector/4 -> HTG/5, Multi-Band Power System Stabilizer/1  "<Rotor speed deviation  dw (pu)>"
  Bus Selector/3 -> HTG/3  "<Rotor speed  wm  (pu)>"
  Pref/1 -> HTG/2
  wref/1 -> HTG/1
  HTG/1 -> Pm/1, Sum2/2
  Bus Selector/2 -> EXCITATION/3  "<Stator voltage  vq (pu)>"
  EXCITATION/1 -> Vf/1
  Bus Selector/1 -> EXCITATION/2  "<Stator voltage  vd (pu)>"
  Sum2/1 -> Generic Power System Stabilizer/1  "Pa = Pm-Pe"
  Generic Power System Stabilizer/1 -> Multiport Switch/3
  Multi-Band Power System Stabilizer/1 -> Multiport Switch/4
  no PSS/1 -> Multiport Switch/2
  Multiport Switch/1 -> EXCITATION/4
  [PSS] -> Sum/1
  PSS/1 -> Sum/2
  Sum/1 -> Multiport Switch/1
  Bus Selector/5 -> Sum2/1, HTG/4  "<Output active power   Peo (pu)>"

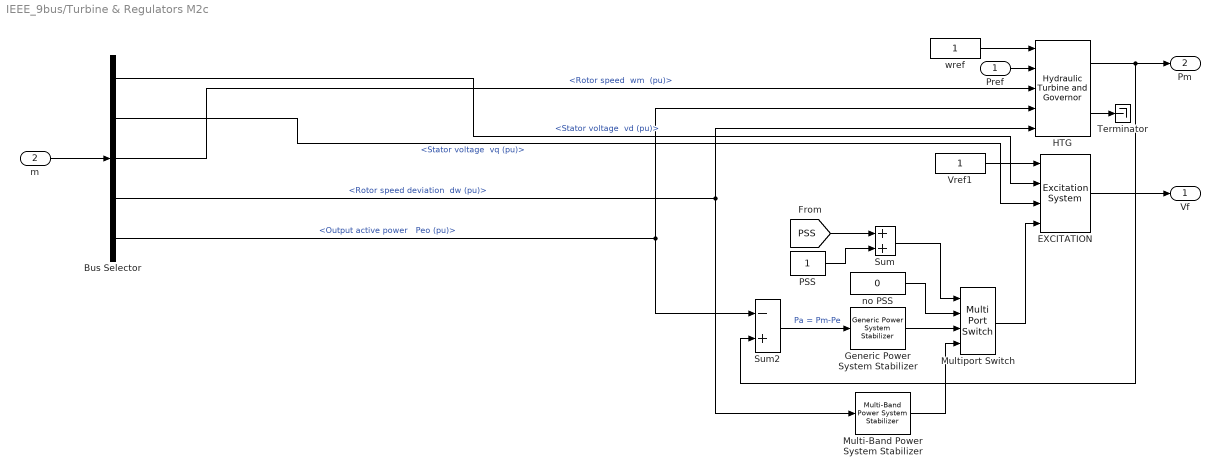
== system IEEE_9bus/Turbine & Regulators M2c ==
  Pref : Inport
  m : Inport  Port=2
  Bus Selector : BusSelector  OutputSignals="Stator voltage  vd (pu),Stator voltage  vq (pu),Rotor speed  wm  (pu),Rotor speed deviation  dw (pu),Output active power   Peo (pu)"
  EXCITATION : spsExcitationSystemLib/Excitation System  tr=20e-3  reg=[ 200, 0.001 ]  exc=[ 1, 0 ]  tgr=[ 0, 0 ]  damp=[ 0.001, 0.1 ]  sat=[ 0, 0 ]  lim="[ 0,  7, 0 ]"  v0=[1 1.5762]
      settings: LibrarySourceBlock=sps_lib/Electrical Machines/Synchronous Machine Control/Excitation System
  Generic Power System Stabilizer : spsGenericPowerSystemStabilizerLib/Generic Power System Stabilizer  Tsensor=15e-3  K=2  Twashout=0.7  Tleadlag1="[60e-3  0.5]"  Tleadlag2=[0 0]  VSlimits=[-0.15 0.15]  Vinit=0  Plot_On=off  MagdB_On=on  FreqRange=logspace(-2,2,500)
      settings: LibrarySourceBlock=|
      | sps_lib/Electrical Machines/Synchronous Machine Control/Generic
      | Power System Stabilizer
  HTG : spsHydraulicTurbineandGovernorLib/Hydraulic Turbine and Governor  sm="[ 10/3  0.07 ]"  gate="[  0.01  0.97518  -0.1  0.1 ]"  reg="[  0.05  1.163  0.105  0  0.01  ]"  hyd="[  0  2.67  ]"  dref=0  po=0.82708
      settings: LibrarySourceBlock=|
      | sps_lib/Electrical Machines/Synchronous Machine Control/Hydraulic Turbine
      | and Governor
  Multi-Band Power System Stabilizer : spsMultiBandPowerSystemStabilizerLib/Multi-Band Power System Stabilizer  OperationMode=Simplified settings  Kg=1.0  GL=[0.025 5]  GI=[0.8 25]  GH=[12.0 145]  GLd=[66 66 9.4]  TcLF=[1.667 2 0 0 0 0 2 2.4 0 0 0 0 1 1]  GId=[66 66 47.6]  TcIF=[1 1 0.25 0.3 0 0 1 1 0.3 0.36 0 0 0 0]  GHd=[66 66 233]  TcHF="[0.01 0.012 0 0 0 0  0.012 0.0144 0 0 0 0 1 1]"  LIM=[.075 .15 .15 .15]  Plot_On=off  MagdB_On=off  FreqRange=logspace(-2,2,500)
      settings: LibrarySourceBlock=|
      | sps_lib/Electrical Machines/Synchronous Machine Control/Multi-Band
      | Power System Stabilizer
  Multiport Switch : MultiPortSwitch  InputSameDT=off
  PSS : Constant
  Sum : Sum  SaturateOnIntegerOverflow=on
  Sum2 : Sum  Inputs=-+  InputSameDT=on  SaturateOnIntegerOverflow=on  OutDataTypeStr=Inherit: Same as first input
  Terminator : Terminator
  Vref1 : Constant
  no PSS : Constant  Value=0
  wref : Constant
  Vf : Outport  InitialOutput=0  VectorParamsAs1DForOutWhenUnconnected=off
  Pm : Outport  Port=2  InitialOutput=0  VectorParamsAs1DForOutWhenUnconnected=off
  wires:
  HTG/2 -> Terminator/1
  Vref1/1 -> EXCITATION/1
  m/1 -> Bus Selector/1
  Bus Selector/4 -> Multi-Band Power System Stabilizer/1, HTG/5  "<Rotor speed deviation  dw (pu)>"
  Bus Selector/3 -> HTG/3  "<Rotor speed  wm  (pu)>"
  Pref/1 -> HTG/2
  wref/1 -> HTG/1
  HTG/1 -> Pm/1, Sum2/2
  Bus Selector/2 -> EXCITATION/3  "<Stator voltage  vq (pu)>"
  EXCITATION/1 -> Vf/1
  Bus Selector/1 -> EXCITATION/2  "<Stator voltage  vd (pu)>"
  Sum2/1 -> Generic Power System Stabilizer/1  "Pa = Pm-Pe"
  Generic Power System Stabilizer/1 -> Multiport Switch/3
  Multi-Band Power System Stabilizer/1 -> Multiport Switch/4
  no PSS/1 -> Multiport Switch/2
  Multiport Switch/1 -> EXCITATION/4
  [PSS] -> Sum/1
  PSS/1 -> Sum/2
  Sum/1 -> Multiport Switch/1
  Bus Selector/5 -> HTG/4, Sum2/1  "<Output active power   Peo (pu)>"

== system IEEE_9bus/Turbine & Regulators M3 ==
  m : Inport
  Pref : Inport  Port=2
  Bus Selector : BusSelector  OutputSignals="dq0 components.Stator voltage  vd (pu),dq0 components.Stator voltage  vq (pu),Mechanical.Rotor speed  wm  (pu),Mechanical.Rotor speed deviation  dw (pu),Output active power   Peo (pu)"
  EXCITATION : spsExcitationSystemLib/Excitation System  tr=20e-3  reg=[ 200, 0.001 ]  exc=[ 1, 0 ]  tgr=[ 0, 0 ]  damp=[ 0.001, 0.1 ]  sat=[ 0, 0 ]  lim="[ 0,  7, 0 ]"  v0=[1 1.2604]
      settings: LibrarySourceBlock=sps_lib/Electrical Machines/Synchronous Machine Control/Excitation System
  Generic Power System Stabilizer : spsGenericPowerSystemStabilizerLib/Generic Power System Stabilizer  Tsensor=15e-3  K=2  Twashout=0.7  Tleadlag1="[60e-3  0.5]"  Tleadlag2=[0 0]  VSlimits=[-0.15 0.15]  Vinit=0  Plot_On=off  MagdB_On=on  FreqRange=logspace(-2,2,500)
      settings: LibrarySourceBlock=|
      | sps_lib/Electrical Machines/Synchronous Machine Control/Generic
      | Power System Stabilizer
  HTG : spsHydraulicTurbineandGovernorLib/Hydraulic Turbine and Governor  sm="[ 10/3  0.07 ]"  gate="[  0.01  0.97518  -0.1  0.1 ]"  reg="[  0.05  1.163  0.105  0  0.01  ]"  hyd="[  0  2.67  ]"  dref=0  po=0.42557
      settings: LibrarySourceBlock=|
      | sps_lib/Electrical Machines/Synchronous Machine Control/Hydraulic Turbine
      | and Governor
  Multi-Band Power System Stabilizer : spsMultiBandPowerSystemStabilizerLib/Multi-Band Power System Stabilizer  OperationMode=Simplified settings  Kg=1.0  GL=[0.025 5]  GI=[0.8 25]  GH=[12.0 145]  GLd=[66 66 9.4]  TcLF=[1.667 2 0 0 0 0 2 2.4 0 0 0 0 1 1]  GId=[66 66 47.6]  TcIF=[1 1 0.25 0.3 0 0 1 1 0.3 0.36 0 0 0 0]  GHd=[66 66 233]  TcHF="[0.01 0.012 0 0 0 0  0.012 0.0144 0 0 0 0 1 1]"  LIM=[.075 .15 .15 .15]  Plot_On=off  MagdB_On=off  FreqRange=logspace(-2,2,500)
      settings: LibrarySourceBlock=|
      | sps_lib/Electrical Machines/Synchronous Machine Control/Multi-Band
      | Power System Stabilizer
  Multiport Switch : MultiPortSwitch  InputSameDT=off
  PSS : Constant
  Sum : Sum  SaturateOnIntegerOverflow=on
  Sum2 : Sum  Inputs=-+  InputSameDT=on  SaturateOnIntegerOverflow=on  OutDataTypeStr=Inherit: Same as first input
  Terminator : Terminator
  Vref1 : Constant
  no PSS : Constant  Value=0
  wref : Constant
  Pm : Outport  InitialOutput=0  VectorParamsAs1DForOutWhenUnconnected=off
  Vf : Outport  Port=2  InitialOutput=0  VectorParamsAs1DForOutWhenUnconnected=off
  wires:
  HTG/2 -> Terminator/1
  Vref1/1 -> EXCITATION/1
  m/1 -> Bus Selector/1
  Bus Selector/4 -> HTG/5, Multi-Band Power System Stabilizer/1  "<Rotor speed deviation  dw (pu)>"
  Bus Selector/3 -> HTG/3  "<Rotor speed  wm  (pu)>"
  Pref/1 -> HTG/2
  wref/1 -> HTG/1
  HTG/1 -> Pm/1, Sum2/2
  Bus Selector/2 -> EXCITATION/3  "<Stator voltage  vq (pu)>"
  EXCITATION/1 -> Vf/1
  Bus Selector/1 -> EXCITATION/2  "<Stator voltage  vd (pu)>"
  Sum2/1 -> Generic Power System Stabilizer/1  "Pa = Pm-Pe"
  Generic Power System Stabilizer/1 -> Multiport Switch/3
  Multi-Band Power System Stabilizer/1 -> Multiport Switch/4
  no PSS/1 -> Multiport Switch/2
  Multiport Switch/1 -> EXCITATION/4
  [PSS] -> Sum/1
  PSS/1 -> Sum/2
  Sum/1 -> Multiport Switch/1
  Bus Selector/5 -> Sum2/1, HTG/4  "<Output active power   Peo (pu)>"

== system IEEE_9bus/Turbine & Regulators M3c ==
  Pref : Inport
  m : Inport  Port=2
  Bus Selector : BusSelector  OutputSignals="Stator voltage  vd (pu),Stator voltage  vq (pu),Rotor speed  wm  (pu),Rotor speed deviation  dw (pu),Output active power   Peo (pu)"
  EXCITATION : spsExcitationSystemLib/Excitation System  tr=20e-3  reg=[ 200, 0.001 ]  exc=[ 1, 0 ]  tgr=[ 0, 0 ]  damp=[ 0.001, 0.1 ]  sat=[ 0, 0 ]  lim="[ 0,  7, 0 ]"  v0=[1 1.2604]
      settings: LibrarySourceBlock=sps_lib/Electrical Machines/Synchronous Machine Control/Excitation System
  Generic Power System Stabilizer : spsGenericPowerSystemStabilizerLib/Generic Power System Stabilizer  Tsensor=15e-3  K=2  Twashout=0.7  Tleadlag1="[60e-3  0.5]"  Tleadlag2=[0 0]  VSlimits=[-0.15 0.15]  Vinit=0  Plot_On=off  MagdB_On=on  FreqRange=logspace(-2,2,500)
      settings: LibrarySourceBlock=|
      | sps_lib/Electrical Machines/Synchronous Machine Control/Generic
      | Power System Stabilizer
  HTG : spsHydraulicTurbineandGovernorLib/Hydraulic Turbine and Governor  sm="[ 10/3  0.07 ]"  gate="[  0.01  0.97518  -0.1  0.1 ]"  reg="[  0.05  1.163  0.105  0  0.01  ]"  hyd="[  0  2.67  ]"  dref=0  po=0.42557
      settings: LibrarySourceBlock=|
      | sps_lib/Electrical Machines/Synchronous Machine Control/Hydraulic Turbine
      | and Governor
  Multi-Band Power System Stabilizer : spsMultiBandPowerSystemStabilizerLib/Multi-Band Power System Stabilizer  OperationMode=Simplified settings  Kg=1.0  GL=[0.025 5]  GI=[0.8 25]  GH=[12.0 145]  GLd=[66 66 9.4]  TcLF=[1.667 2 0 0 0 0 2 2.4 0 0 0 0 1 1]  GId=[66 66 47.6]  TcIF=[1 1 0.25 0.3 0 0 1 1 0.3 0.36 0 0 0 0]  GHd=[66 66 233]  TcHF="[0.01 0.012 0 0 0 0  0.012 0.0144 0 0 0 0 1 1]"  LIM=[.075 .15 .15 .15]  Plot_On=off  MagdB_On=off  FreqRange=logspace(-2,2,500)
      settings: LibrarySourceBlock=|
      | sps_lib/Electrical Machines/Synchronous Machine Control/Multi-Band
      | Power System Stabilizer
  Multiport Switch : MultiPortSwitch  InputSameDT=off
  PSS : Constant
  Sum : Sum  SaturateOnIntegerOverflow=on
  Sum2 : Sum  Inputs=-+  InputSameDT=on  SaturateOnIntegerOverflow=on  OutDataTypeStr=Inherit: Same as first input
  Terminator : Terminator
  Vref1 : Constant
  no PSS : Constant  Value=0
  wref : Constant
  Pm : Outport  InitialOutput=0  VectorParamsAs1DForOutWhenUnconnected=off
  Vf : Outport  Port=2  InitialOutput=0  VectorParamsAs1DForOutWhenUnconnected=off
  wires:
  HTG/2 -> Terminator/1
  Vref1/1 -> EXCITATION/1
  m/1 -> Bus Selector/1
  Bus Selector/4 -> HTG/5, Multi-Band Power System Stabilizer/1  "<Rotor speed deviation  dw (pu)>"
  Bus Selector/3 -> HTG/3  "<Rotor speed  wm  (pu)>"
  Pref/1 -> HTG/2
  wref/1 -> HTG/1
  HTG/1 -> Pm/1, Sum2/2
  Bus Selector/2 -> EXCITATION/3  "<Stator voltage  vq (pu)>"
  EXCITATION/1 -> Vf/1
  Bus Selector/1 -> EXCITATION/2  "<Stator voltage  vd (pu)>"
  Sum2/1 -> Generic Power System Stabilizer/1  "Pa = Pm-Pe"
  Generic Power System Stabilizer/1 -> Multiport Switch/3
  Multi-Band Power System Stabilizer/1 -> Multiport Switch/4
  no PSS/1 -> Multiport Switch/2
  Multiport Switch/1 -> EXCITATION/4
  [PSS] -> Sum/1
  PSS/1 -> Sum/2
  Sum/1 -> Multiport Switch/1
  Bus Selector/5 -> HTG/4, Sum2/1  "<Output active power   Peo (pu)>"

== system IEEE_9bus/DQN_Mac1_V1/ABsel2 ==
  v : Inport
  Demux : Demux  Outputs=2
  Mux : Mux  Inputs=3
  Subtract : Sum  Inputs=--
  I : Outport
  wires:
  v/1 -> Demux/1
  Mux/1 -> I/1
  Demux/1 -> Subtract/1, Mux/1
  Demux/2 -> Subtract/2, Mux/2
  Subtract/1 -> Mux/3

== system IEEE_9bus/DQN_Mac1_V1/ABsel3 ==
  v : Inport
  Demux : Demux  Outputs=3
  Mux : Mux  Inputs=2
  Subtract : Sum  Inputs=+-
  Subtract1 : Sum  Inputs=+-
  Out1 : Outport
  wires:
  v/1 -> Demux/1
  Mux/1 -> Out1/1
  Demux/1 -> Subtract/1
  Demux/2 -> Subtract1/1, Subtract/2
  Subtract/1 -> Mux/1
  Subtract1/1 -> Mux/2
  Demux/3 -> Subtract1/2

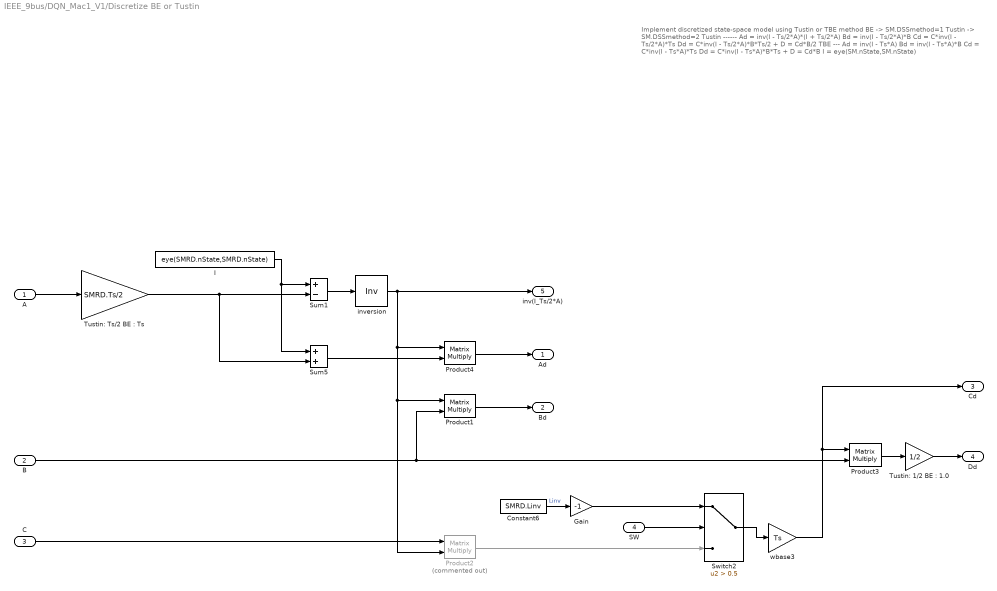
== system IEEE_9bus/DQN_Mac1_V1/Discretize BE or Tustin ==
  note: Implement discretized state-space model using Tustin or TBE method
      |
      | BE      -> SM.DSSmethod=1
      | Tustin  -> SM.DSSmethod=2
      |
      |
      | Tustin
      | ------
      | Ad = inv(I - Ts/2*A)*(I + Ts/2*A)
      | Bd = inv(I - Ts/2*A)*B
      | Cd = C*inv(I - Ts/2*A)*Ts
      | Dd = C*inv(I - Ts/2*A)*B*Ts/2  + D  =  Cd*B/2
      |
      | TBE
      | ---
      | Ad = inv(I - Ts*A)
      | Bd = inv(I - Ts*A)*B
      | Cd = C*inv(I - Ts*A)*Ts
      | Dd = C*inv(I - Ts*A)*B*Ts  + D  =  Cd*B
      |
      | I = eye(SM.nState,SM.nState)
  A : Inport
  B : Inport  Port=2
  C : Inport  Port=3
  SW : Inport  Port=4
  Constant6 : Constant  Value=SMRD.Linv
  Gain : Gain  Gain=-1
  I : Constant  Value=eye(SMRD.nState,SMRD.nState)
  Product1 : Product  Multiplication=Matrix(*)  SaturateOnIntegerOverflow=on  OutDataTypeStr=Inherit: Same as first input
  Product2 : Product  Commented=on  Multiplication=Matrix(*)  SaturateOnIntegerOverflow=on  OutDataTypeStr=Inherit: Same as first input
  Product3 : Product  Multiplication=Matrix(*)  SaturateOnIntegerOverflow=on  OutDataTypeStr=Inherit: Same as first input
  Product4 : Product  Multiplication=Matrix(*)  SaturateOnIntegerOverflow=on  OutDataTypeStr=Inherit: Same as first input
  Sum1 : Sum  Inputs=+-  SaturateOnIntegerOverflow=on
  Sum5 : Sum  SaturateOnIntegerOverflow=on
  Switch2 : Switch  Criteria=u2 > Threshold  Threshold=0.5  SaturateOnIntegerOverflow=off  InputSameDT=off
  "Tustin: 1/2 BE : 1.0" : Gain  Gain=1/2  SaturateOnIntegerOverflow=on  OutDataTypeStr=Inherit: Same as input  ParamDataTypeStr=Inherit: Same as input
  "Tustin: Ts/2 BE : Ts" : Gain  Gain=SMRD.Ts/2  SaturateOnIntegerOverflow=on  OutDataTypeStr=Inherit: Same as input  ParamDataTypeStr=Inherit: Same as input
  inversion : Product  Inputs=/  Multiplication=Matrix(*)  RndMeth=Zero
  wbase3 : Gain  Gain=Ts  SaturateOnIntegerOverflow=on  OutDataTypeStr=Inherit: Same as input  ParamDataTypeStr=Inherit: Same as input
  Ad : Outport  VectorParamsAs1DForOutWhenUnconnected=off
  Bd : Outport  Port=2  VectorParamsAs1DForOutWhenUnconnected=off
  Cd : Outport  Port=3  VectorParamsAs1DForOutWhenUnconnected=off
  Dd : Outport  Port=4  VectorParamsAs1DForOutWhenUnconnected=off
  inv(I_Ts/2*A) : Outport  Port=5  VectorParamsAs1DForOutWhenUnconnected=off
  wires:
  "Tustin: Ts/2 BE : Ts"/1 -> Sum1/2, Sum5/2
  Product4/1 -> Ad/1
  A/1 -> "Tustin: Ts/2 BE : Ts"/1
  I/1 -> Sum5/1, Sum1/1
  Sum1/1 -> inversion/1
  inversion/1 -> Product2/2, Product1/1, Product4/1, inv(I_Ts/2*A)/1
  Sum5/1 -> Product4/2
  Product1/1 -> Bd/1
  B/1 -> Product1/2, Product3/2
  C/1 -> Product2/1
  Product3/1 -> "Tustin: 1/2 BE : 1.0"/1
  "Tustin: 1/2 BE : 1.0"/1 -> Dd/1
  Switch2/1 -> wbase3/1
  Constant6/1 -> Gain/1  "Linv"
  SW/1 -> Switch2/2
  Product2/1 -> Switch2/3
  wbase3/1 -> Cd/1, Product3/1
  Gain/1 -> Switch2/1

== system IEEE_9bus/DQN_Mac1_V1/Electromagnetic Torque ==
  note: Te computed from stator fluxes and currents
  note: Te=phids*Iqs - phiqs*Ids
  phiqd : Inport
  iqd : Inport  Port=2
  1-1 : Gain  Gain=[1 -1]
  Mult1 : Product  Inputs=**
  Selector1 : Selector  InputPortWidth=2  IndexOptions=Index vector (dialog)  Indices="[2  1]"  OutputSizes=1
  Sum2 : Sum  Inputs=1  SaturateOnIntegerOverflow=on
  Te : Outport  VectorParamsAs1DForOutWhenUnconnected=off
  wires:
  Mult1/1 -> Sum2/1
  1-1/1 -> Mult1/2  "iqs -ids"
  Selector1/1 -> Mult1/1  "phids phiqs"
  Sum2/1 -> Te/1
  phiqd/1 -> Selector1/1
  iqd/1 -> 1-1/1

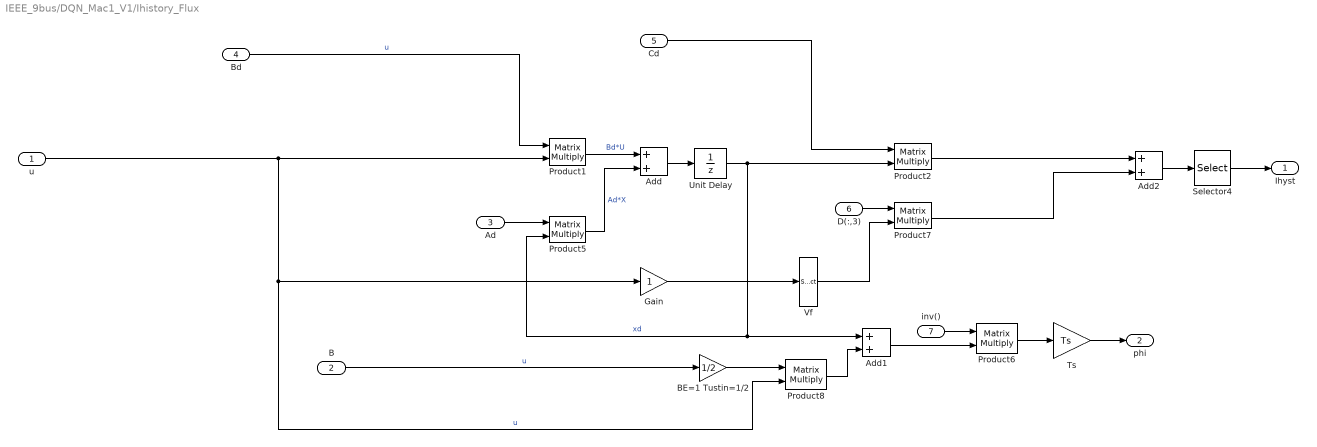
== system IEEE_9bus/DQN_Mac1_V1/Ihistory_Flux ==
  u : Inport
  B : Inport  Port=2
  Ad : Inport  Port=3
  Bd : Inport  Port=4
  Cd : Inport  Port=5
  D(:,3) : Inport  Port=6
  inv() : Inport  Port=7
  Add : Sum
  Add1 : Sum
  Add2 : Sum
  BE=1 Tustin=1/2 : Gain  Gain=1/2
  Gain : Gain
  Product{1..2,5..8} (6 alike) : Product  Multiplication=Matrix(*)  SaturateOnIntegerOverflow=on  OutDataTypeStr=Inherit: Same as first input
  Selector4 : Selector  InputPortWidth=SMRD.nState  IndexOptions=Index vector (dialog)  Indices=[1 2]  OutputSizes=1
  Ts : Gain  Gain=Ts  SaturateOnIntegerOverflow=on  OutDataTypeStr=Inherit: Same as input  ParamDataTypeStr=Inherit: Same as input
  Unit Delay : UnitDelay  InitialCondition=SMRD.phidq0/Ts  SampleTime=Ts  HasFrameUpgradeWarning=on
  Vf : Selector  InputPortWidth=SMRD.nState  IndexOptions=Index vector (dialog)  Indices=3  OutputSizes=1
  Ihyst : Outport  VectorParamsAs1DForOutWhenUnconnected=off
  phi : Outport  Port=2  VectorParamsAs1DForOutWhenUnconnected=off
  wires:
  BE=1 Tustin=1/2/1 -> Product8/1
  inv()/1 -> Product6/1
  Cd/1 -> Product2/1
  Ad/1 -> Product5/1
  Add1/1 -> Product6/2
  Product8/1 -> Add1/2
  Product6/1 -> Ts/1
  Product5/1 -> Add/2  "Ad*X"
  Unit Delay/1 -> Product5/2, Add1/1, Product2/2  "xd"
  Add/1 -> Unit Delay/1
  Product1/1 -> Add/1  "Bd*U"
  Product2/1 -> Add2/1
  Add2/1 -> Selector4/1
  Product7/1 -> Add2/2
  Vf/1 -> Product7/2
  D(:,3)/1 -> Product7/1
  u/1 -> Product1/2, Gain/1, Product8/2  "u"
  Bd/1 -> Product1/1  "u"
  B/1 -> BE=1 Tustin=1/2/1  "u"
  Selector4/1 -> Ihyst/1
  Gain/1 -> Vf/1
  Ts/1 -> phi/1

== system IEEE_9bus/DQN_Mac1_V1/Matrix W ==
  wr : Inport
  Gain1 : Gain  Gain=-1  SaturateOnIntegerOverflow=on  OutDataTypeStr=Inherit: Same as input  ParamDataTypeStr=Inherit: Same as input
  W(1,2)=wr : Assignment  NumberOfDimensions=2  IndexOptions=Index vector (dialog),Index vector (dialog)  Indices=1,2  OutputSizes=1,1
  W(2,1)=-wr : Assignment  NumberOfDimensions=2  IndexOptions=Index vector (dialog),Index vector (dialog)  Indices=2,1  OutputSizes=1,1
  u1 : Constant  Value=zeros(SMRD.nState,SMRD.nState)
  "[W]" : Outport  VectorParamsAs1DForOutWhenUnconnected=off
  wires:
  u1/1 -> W(1,2)=wr/1
  Gain1/1 -> W(2,1)=-wr/2
  W(1,2)=wr/1 -> W(2,1)=-wr/1
  wr/1 -> W(1,2)=wr/2, Gain1/1
  W(2,1)=-wr/1 -> "[W]"/1

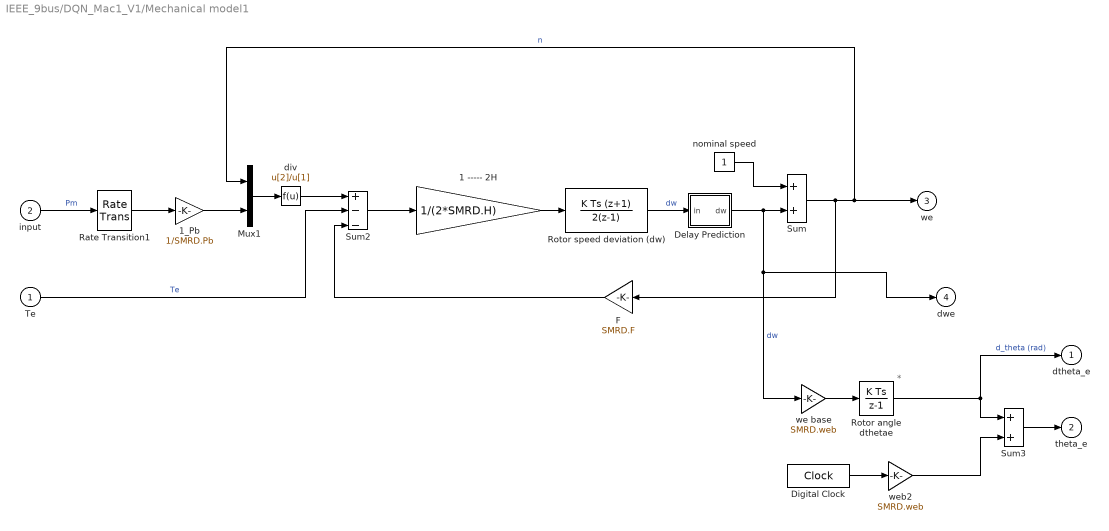
== system IEEE_9bus/DQN_Mac1_V1/Mechanical model1 ==
  note: *
  Te : Inport  PortDimensions=1
  input : Inport  Port=2
  1 ----- 2H : Gain  Gain=1/(2*SMRD.H)  SaturateOnIntegerOverflow=on  OutDataTypeStr=Inherit: Same as input  ParamDataTypeStr=Inherit: Same as input
  1_Pb : Gain  Gain=1/SMRD.Pb  SaturateOnIntegerOverflow=on  OutDataTypeStr=Inherit: Same as input  ParamDataTypeStr=Inherit: Same as input
  Delay Prediction : Subsystem
  Digital Clock : DigitalClock  SampleTime=SMRD.Ts
  F : Gain  Gain=SMRD.F  SaturateOnIntegerOverflow=on  OutDataTypeStr=Inherit: Same as input  ParamDataTypeStr=Inherit: Same as input
  Mux1 : Mux  Inputs=2
  Rate Transition1 : RateTransition  Deterministic=off  OutPortSampleTime=Ts
  Rotor angle dthetae : DiscreteIntegrator  InitialCondition=SMRD.tho  SampleTime=SMRD.Ts  ICPrevOutput=DiscIntNeverNeededParam  ICPrevScaledInput=DiscIntNeverNeededParam
  Rotor speed deviation (dw) : DiscreteIntegrator  IntegratorMethod=Integration: Trapezoidal  InitialCondition=SMRD.dwo  SampleTime=SMRD.Ts  ICPrevOutput=DiscIntNeverNeededParam  ICPrevScaledInput=DiscIntNeverNeededParam
  Sum : Sum  InputSameDT=on  SaturateOnIntegerOverflow=on  OutDataTypeStr=Inherit: Same as first input
  Sum2 : Sum  Inputs=+--  InputSameDT=on  SaturateOnIntegerOverflow=on  OutDataTypeStr=Inherit: Same as first input
  Sum3 : Sum  InputSameDT=on  SaturateOnIntegerOverflow=on  OutDataTypeStr=Inherit: Same as first input
  div : Fcn  Expr=u[2]/u[1]
      mask Display: disp('/')
  nominal speed : Constant
  we base : Gain  Gain=SMRD.web  SaturateOnIntegerOverflow=on  OutDataTypeStr=Inherit: Same as input  ParamDataTypeStr=Inherit: Same as input
  web2 : Gain  Gain=SMRD.web  SaturateOnIntegerOverflow=on  OutDataTypeStr=Inherit: Same as input  ParamDataTypeStr=Inherit: Same as input
  dtheta_e : Outport  InitialOutput=0  VectorParamsAs1DForOutWhenUnconnected=off
  theta_e : Outport  Port=2  InitialOutput=0  VectorParamsAs1DForOutWhenUnconnected=off
  we : Outport  Port=3  InitialOutput=0  VectorParamsAs1DForOutWhenUnconnected=off
  dwe : Outport  Port=4  InitialOutput=0  VectorParamsAs1DForOutWhenUnconnected=off
  wires:
  Delay Prediction/1(dw) -> dwe/1, we base/1, Sum/2  "dw"
  Rate Transition1/1 -> 1_Pb/1
  Rotor angle dthetae/1 -> Sum3/1, dtheta_e/1  "d_theta (rad)"
  web2/1 -> Sum3/2
  Digital Clock/1 -> web2/1
  we base/1 -> Rotor angle dthetae/1
  Rotor speed deviation (dw)/1 -> Delay Prediction/1(in)  "dw"
  nominal speed/1 -> Sum/1
  1 ----- 2H/1 -> Rotor speed deviation (dw)/1
  div/1 -> Sum2/1
  Te/1 -> Sum2/2  "Te"
  Mux1/1 -> div/1
  input/1 -> Rate Transition1/1  "Pm"
  1_Pb/1 -> Mux1/2
  F/1 -> Sum2/3
  Sum2/1 -> 1 ----- 2H/1
  Sum/1 -> F/1, we/1, Mux1/1  "n"
  Sum3/1 -> theta_e/1
